simulink model "drone_altitude_control_sim"  (R2023b)
settings: Solver=VariableStepAuto  StartTime=0.0  StopTime=1000  RelTol=1e-3
values from neighbouring files (symbols this model uses):
  d = 0.5    [drone_altitude_control.m]
  g = 9.81    [drone_altitude_control.m]
  KD = 0.17    [drone_altitude_control.m]
  KI = 0.001    [drone_altitude_control.m]
  KP = 0.07    [drone_altitude_control.m]
  m = 1.5    [drone_altitude_control.m]
libraries: simulink x1
settings Model: Creator=user  LastModifiedBy=user

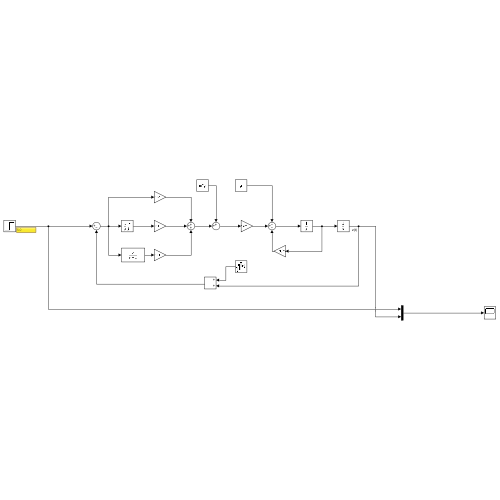
[thumbnail: Simulink's stored preview of the top-level diagram]
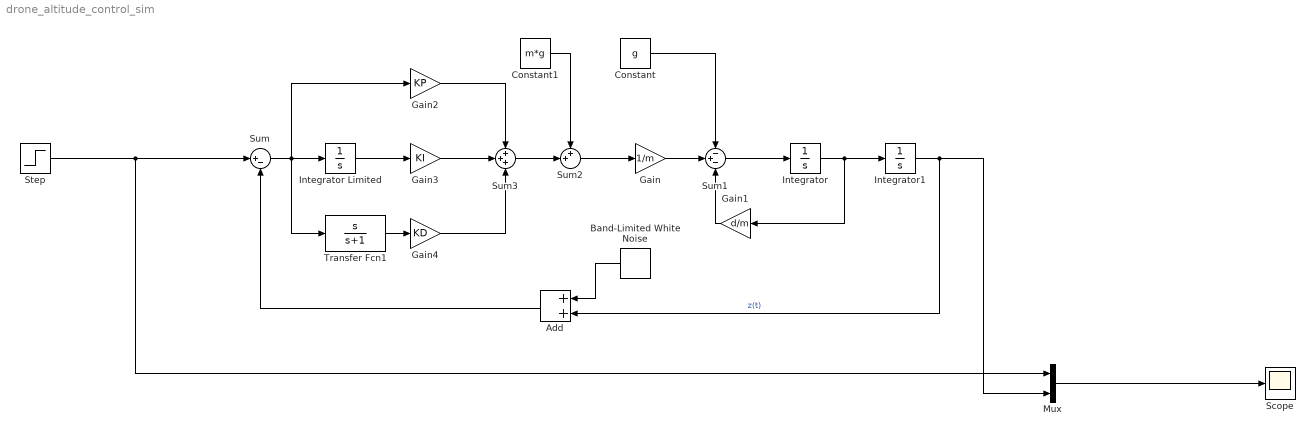
== system drone_altitude_control_sim ==
  Add : Sum
  Band-Limited White Noise : simulink/Sources/Band-Limited White Noise  Cov=[0.5]  Ts=0.01  seed=[23341]
  Constant : Constant  Value=g
  Constant1 : Constant  Value=m*g
  Gain : Gain  Gain=1/m
  Gain1 : Gain  Gain=d/m
  Gain2 : Gain  Gain=KP
  Gain3 : Gain  Gain=KI
  Gain4 : Gain  Gain=KD
  Integrator : Integrator
  Integrator Limited : Integrator  LimitOutput=on  UpperSaturationLimit=15  LowerSaturationLimit=0
  Integrator1 : Integrator
  Mux : Mux  Inputs=2
  Scope : Scope
  Step : Step  After=50  SampleTime=0
  Sum : Sum  Inputs=|+-
  Sum1 : Sum  Inputs=-+-
  Sum2 : Sum  Inputs=++|
  Sum3 : Sum  Inputs=+++
  Transfer Fcn1 : TransferFcn  Numerator=[1 0]  Denominator=[1 1]
  wires:
  Integrator1/1 -> Add/2, Mux/2  "z(t)"
  Mux/1 -> Scope/1
  Gain/1 -> Sum1/2
  Constant/1 -> Sum1/1
  Sum1/1 -> Integrator/1
  Integrator/1 -> Gain1/1, Integrator1/1
  Gain1/1 -> Sum1/3
  Constant1/1 -> Sum2/1
  Sum2/1 -> Gain/1
  Step/1 -> Mux/1, Sum/1
  Sum/1 -> Transfer Fcn1/1, Integrator Limited/1, Gain2/1
  Sum3/1 -> Sum2/2
  Band-Limited White Noise/1 -> Add/1
  Add/1 -> Sum/2
  Gain3/1 -> Sum3/2
  Gain2/1 -> Sum3/1
  Gain4/1 -> Sum3/3
  Integrator Limited/1 -> Gain3/1
  Transfer Fcn1/1 -> Gain4/1
